simulink model "KVHSerial03"  (R2013a)
settings: Solver=FixedStepDiscrete  StartTime=0.0  StopTime=inf  FixedStep=0.001  RelTol=1e-3
undefined symbols (not defined in the file or in its folder): Ground, m_XR17D15x, standard, XOFF, XON
libraries: speedgoatlib x26, xpcseriallib x13, simulink x3, xpclib x2
settings Model: BufferReuse=off  Creator=bgbuss  LastModifiedBy=bgbuss
settings DataIOCC: LimitDataPoints=off  SignalLoggingSaveFormat=ModelDataLogs
settings OptimizationCC: BlockReduction=off  OptimizeBlockIOStorage=off  BufferReuse=off  ExpressionFolding=off  ExpressionDepthLimit=2147483647  LocalBlockOutputs=off
settings DebuggingCC: UnderspecifiedInitializationDetection=Simplified  FcnCallInpInsideContextMsg=EnableAllAsWarning  StrictBusMsg=ErrorOnBusTreatedAsVector
settings HardwareCC: ProdIntDivRoundTo=Zero  ProdEndianess=LittleEndian  ProdHWDeviceType=Generic->32-bit x86 compatible
settings RTWCC: SystemTargetFile=xpctarget.tlc  TemplateMakefile=xpc_default_tmf  Description=xPC Target  ProcessScript=xpctarget_make_rtw_hook
settings xpcTargetCC: TargetFcnLib=ansi_tfl_table_tmw.mat  CodeReplacementLibrary=XPC_BLAS  ParMdlRefBuildCompliant=on  ConcurrentExecutionCompliant=on  CombineSignalStateStructs=off  MATLABClassNameForMDSCustomization=xpcAperiodicCustomization  GRTInterface=on  GenerateAllocFcn=off  RL32LogBufSizeModifier=10000000  xPCTaskExecutionProfile=off  xPCRL32EventNumber=5000  xPCisModelTimeout=off  xPCModelTimeoutSecs=10  xPCLoadParamSetFile=off  xPCConcurrentTasks=off  xPCEnableSFAnimation=off

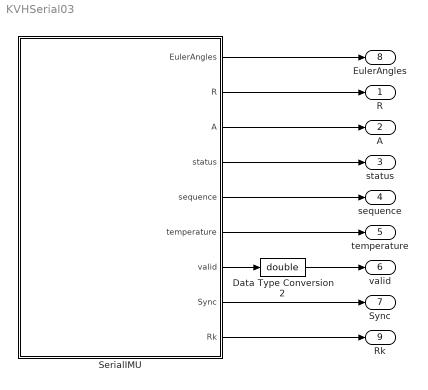
== system KVHSerial03 ==
  Data Type Conversion2 : DataTypeConversion  OutDataTypeStr=double
  SerialIMU : Subsystem
  R : Outport
  A : Outport  Port=2
  status : Outport  Port=3
  sequence : Outport  Port=4
  temperature : Outport  Port=5
  valid : Outport  Port=6
  Sync : Outport  Port=7
  EulerAngles : Outport  Port=8
  Rk : Outport  Port=9
  wires:
  SerialIMU/7(valid) -> Data Type Conversion2/1
  SerialIMU/3(A) -> A/1
  SerialIMU/2(R) -> R/1
  SerialIMU/4(status) -> status/1
  SerialIMU/5(sequence) -> sequence/1
  SerialIMU/6(temperature) -> temperature/1
  SerialIMU/8(Sync) -> Sync/1
  SerialIMU/1(EulerAngles) -> EulerAngles/1
  SerialIMU/9(Rk) -> Rk/1
  Data Type Conversion2/1 -> valid/1

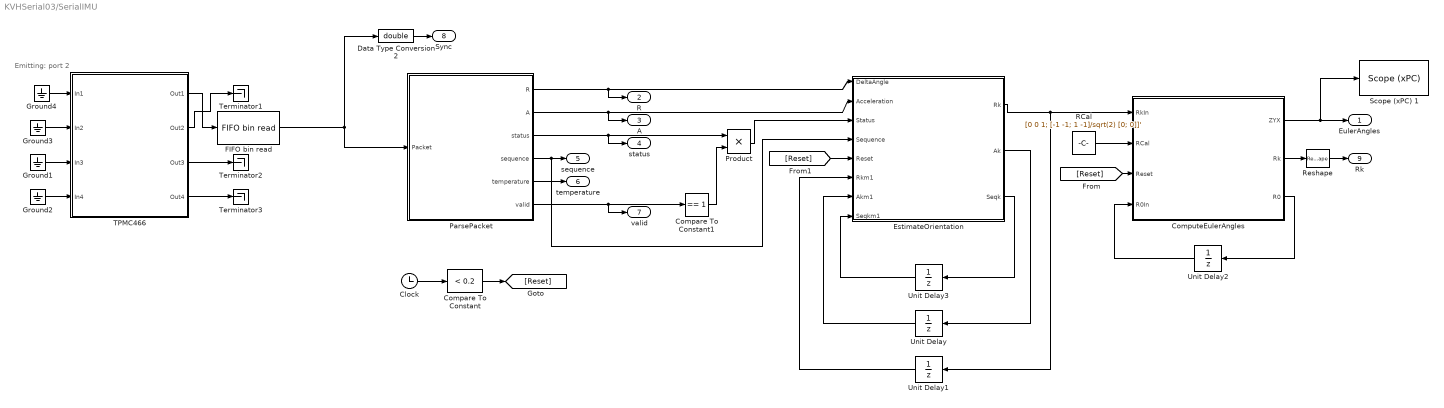
== system KVHSerial03/SerialIMU ==
  note: Emitting: port 2
  Clock : Clock
  Compare To Constant : simulink/Logic and Bit Operations/Compare To Constant  relop=<  const=0.2  OutDataTypeStr=uint8
  Compare To Constant1 : simulink/Logic and Bit Operations/Compare To Constant  relop===  const=1  OutDataTypeStr=uint8
  ComputeEulerAngles : MATLAB Function  TreatAsAtomicUnit=on
  Data Type Conversion2 : DataTypeConversion  OutDataTypeStr=double
  EstimateOrientation : MATLAB Function  TreatAsAtomicUnit=on
  "FIFO bin read " : xpcseriallib/FIFO bin read   header={char([254 129 255 85])}  lengths=[36]  hold=Zero output if no new data  enable=off  maxsize=64  outputtype=8 bit uint null terminated  sampletime=0.001
  Ground{1..4} (4 alike) : Ground
  ParsePacket : Subsystem
  Product : Product  RndMeth=Zero
  RCal : Constant  Value=[0 0 1; [-1 -1; 1 -1]/sqrt(2) [0; 0]]'
  Reshape : Reshape
  Scope (xPC) 1 : xpclib/Misc./Scope (xPC)   scopeno=1  scopetype=Target  autostart=on  viewmode=Graphical rolling  formatstr='%15.6f'  grid=on  ylimits=[-pi pi]  nosamples=500  noprepostsamples=0  interleave=10  triggermode=FreeRun  triggersignal=1  trigsignalfromport=off  triggerlevel=0.0  triggerslope=Either  triggerscope=1  triggersample=0  filename=data.dat  mode=Lazy  writesize=512  autorestart=off  dynamicfilemode=off  maxwritefilesize=512*1024^2
  TPMC466 : Subsystem  AncestorBlock=speedgoatlib/IO503/TPMC466  InitFcn=m_XR17D15x(3);  mask(RS232 Send Receive){group=Basic Setup, port=1, irqnum=9, slot=-1, transceiver1=RS422, standard1=on, baud1=921600, bauddivisor1=1, sampling1=16x (standard), prescale1=off, parity1=None, ndata1=8, nstop1=1, rlevel1=1, hwmode1=none, swmode1=none, xonchar1=17, xoffchar1=19, rs485auto1=off, rs485delay1=1, xmtfifosize1=1024, xmtdatatype1=8 bit uint null terminated, rcvfifosize1=1024, transceiver2=RS485 half-duplex, standard2=on, baud2=2764800, bauddivisor2=1, sampling2=16x (standard), prescale2=off, parity2=None, ndata2=8, nstop2=1, rlevel2=quarter full (16), hwmode2=none, swmode2=XON/XOFF, xonchar2=17, xoffchar2=19, rs485auto2=on, rs485delay2=1, xmtfifosize2=1024, xmtdatatype2=8 bit uint null terminated, rcvfifosize2=1024, transceiver3=RS485 half-duplex, standard3=on, baud3=115200, bauddivisor3=1, sampling3=16x (standard), prescale3=off, parity3=None, ndata3=8, nstop3=1, rlevel3=half full (32), hwmode3=none, swmode3=none, xonchar3=17, xoffchar3=19, rs485auto3=off, rs485delay3=0, xmtfifosize3=1024, xmtdatatype3=8 bit uint null terminated, rcvfifosize3=1024, transceiver4=RS485 half-duplex, standard4=on, baud4=115200, bauddivisor4=1, sampling4=16x (standard), prescale4=off, parity4=None, ndata4=8, nstop4=1, rlevel4=half full (32), hwmode4=none, swmode4=none, xonchar4=17, xoffchar4=19, rs485auto4=off, rs485delay4=0, xmtfifosize4=1024, xmtdatatype4=8 bit uint null terminated, rcvfifosize4=1024}
      mask prompts: group "Parameter group:"; port "Port to modify:"; irqnum "IRQ number:"; slot "PCI slot (-1: autosearch):"; transceiver1 "Transceiver setup:"; standard1 "Use standard baud rates (16x, no prescaling)"; baud1 "Standard baud rate:"; bauddivisor1 "Baud rate divisor (non-standard baud rates):"; sampling1 "Sampling rate (non-standard baud rates):"; prescale1 "Prescale by 4 (non-standard baud rates)"; parity1 "Parity:"; ndata1 "Data bits:"; nstop1 "Stop bits:"; rlevel1 "Receive FIFO interrupt level:"; hwmode1 "Hardware handshake:"; swmode1 "Software handshake:"; xonchar1 "XON character:"; xoffchar1 "XOFF character:"; rs485auto1 "RS485 auto turnaround:"; rs485delay1 "RS485 turnaround delay [0,15]"; xmtfifosize1 "Transmit software FIFO size:"; xmtdatatype1 "Transmit FIFO data type:"; rcvfifosize1 "Receive software FIFO size:"; transceiver2 "Transceiver setup:"; standard2 "Use standard baud rates (16x, no prescaling)"; baud2 "Standard baud rate:"; bauddivisor2 "Baud rate divisor (non-standard baud rates):"; sampling2 "Sampling rate (non-standard baud rates):"; prescale2 "Prescale by 4 (non-standard baud rates)"; parity2 "Parity:"; ndata2 "Data bits:"; nstop2 "Stop bits:"; rlevel2 "Receive FIFO interrupt level:"; hwmode2 "Hardware handshake:"; swmode2 "Software handshake:"; xonchar2 "XON character:"; xoffchar2 "XOFF character:"; rs485auto2 "RS485 auto turnaround:"; rs485delay2 "RS485 turnaround delay [0,15]"; xmtfifosize2 "Transmit software FIFO size:"; xmtdatatype2 "Transmit FIFO data type:"; rcvfifosize2 "Receive software FIFO size:"; transceiver3 "Transceiver setup:"; standard3 "Use standard baud rates (16x, no prescaling)"; baud3 "Standard baud rate:"; bauddivisor3 "Baud rate divisor (non-standard baud rates):"; sampling3 "Sampling rate (non-standard baud rates):"; prescale3 "Prescale by 4 (non-standard baud rates)"; parity3 "Parity:"; ndata3 "Data bits:"; nstop3 "Stop bits:"; rlevel3 "Receive FIFO interrupt level:"; hwmode3 "Hardware handshake:"; swmode3 "Software handshake:"; xonchar3 "XON character:"; xoffchar3 "XOFF character:"; rs485auto3 "RS485 auto turnaround:"; rs485delay3 "RS485 turnaround delay [0,15]"; xmtfifosize3 "Transmit software FIFO size:"; xmtdatatype3 "Transmit FIFO data type:"; rcvfifosize3 "Receive software FIFO size:"; transceiver4 "Transceiver setup:"; standard4 "Use standard baud rates (16x, no prescaling)"; baud4 "Standard baud rate:"; bauddivisor4 "Baud rate divisor (non-standard baud rates):"; sampling4 "Sampling rate (non-standard baud rates):"; prescale4 "Prescale by 4 (non-standard baud rates)"; parity4 "Parity:"; ndata4 "Data bits:"; nstop4 "Stop bits:"; rlevel4 "Receive FIFO interrupt level:"; hwmode4 "Hardware handshake:"; swmode4 "Software handshake:"; xonchar4 "XON character:"; xoffchar4 "XOFF character:"; rs485auto4 "RS485 auto turnaround:"; rs485delay4 "RS485 turnaround delay [0,15]"; xmtfifosize4 "Transmit software FIFO size:"; xmtdatatype4 "Transmit FIFO data type:"; rcvfifosize4 "Receive software FIFO size:"
      mask help:
      | PMC521
      | Acromag
      | EIA/TIA-422B Send Receive Subsystem
      mask init:
      | brdslot = slot;
      | m_tews_XR17D15x(1, 4);
      mask Help: helpview(fullfile(docroot, 'mapfiles', 'xpc.map'), 'Commtech_Subsystem')
      mask TypeOptions group: Board Setup | Basic Setup | FIFO Setup
      mask Callback group: m_tews_XR17D15x(2, 4);
      mask TypeOptions port: 1 | 2 | 3 | 4
      mask Callback port: m_tews_XR17D15x(2, 4);
      mask TypeOptions transceiver1: RS232 (max 921.6kb/s) | RS422 | RS422 multidrop | RS485 full-duplex | RS485 half-duplex
      mask TypeOptions baud1: 2764800 | 1382400 | 921600 | 460800 | 230400 | 115200 | 57600 | 38400 | 19200 | 9600 | 4800 | 2400 | 1200 | 600 | 400
      mask TypeOptions sampling1: 8x | 16x (standard)
      mask TypeOptions parity1: None | Even | Odd | Mark | Space
      mask TypeOptions ndata1: 5 | 6 | 7 | 8
      mask TypeOptions nstop1: 1 | 2
      mask TypeOptions rlevel1: 1 | quarter full (16) | half full (32) | almost full (56)
      mask TypeOptions hwmode1: RTS/CTS | none
      mask TypeOptions swmode1: XON/XOFF | none
      mask TypeOptions xmtdatatype1: count+32 bit int | count+32 bit uint | count+16 bit int | count+16 bit uint | 8 bit int null terminated | 8 bit uint null terminated
      mask TypeOptions transceiver2: RS232 (max 921.6kb/s) | RS422 | RS422 multidrop | RS485 full-duplex | RS485 half-duplex
      mask TypeOptions baud2: 2764800 | 1382400 | 921600 | 460800 | 230400 | 115200 | 57600 | 38400 | 19200 | 9600 | 4800 | 2400 | 1200 | 600 | 400
      mask TypeOptions sampling2: 8x | 16x (standard)
      mask TypeOptions parity2: None | Even | Odd | Mark | Space
      mask TypeOptions ndata2: 5 | 6 | 7 | 8
      mask TypeOptions nstop2: 1 | 2
      mask TypeOptions rlevel2: 1 | quarter full (16) | half full (32) | almost full (56)
      mask TypeOptions hwmode2: RTS/CTS | none
      mask TypeOptions swmode2: XON/XOFF | none
      mask TypeOptions xmtdatatype2: count+32 bit int | count+32 bit uint | count+16 bit int | count+16 bit uint | 8 bit int null terminated | 8 bit uint null terminated
      mask TypeOptions transceiver3: RS232 (max 921.6kb/s) | RS422 | RS422 multidrop | RS485 full-duplex | RS485 half-duplex
      mask TypeOptions baud3: 2764800 | 1382400 | 921600 | 460800 | 230400 | 115200 | 57600 | 38400 | 19200 | 9600 | 4800 | 2400 | 1200 | 600 | 400
      mask TypeOptions sampling3: 8x | 16x (standard)
      mask TypeOptions parity3: None | Even | Odd | Mark | Space
      mask TypeOptions ndata3: 5 | 6 | 7 | 8
      mask TypeOptions nstop3: 1 | 2
      mask TypeOptions rlevel3: 1 | quarter full (16) | half full (32) | almost full (56)
      mask TypeOptions hwmode3: RTS/CTS | none
      mask TypeOptions swmode3: XON/XOFF | none
      mask TypeOptions xmtdatatype3: count+32 bit int | count+32 bit uint | count+16 bit int | count+16 bit uint | 8 bit int null terminated | 8 bit uint null terminated
      mask TypeOptions transceiver4: RS232 (max 921.6kb/s) | RS422 | RS422 multidrop | RS485 full-duplex | RS485 half-duplex
      mask TypeOptions baud4: 2764800 | 1382400 | 921600 | 460800 | 230400 | 115200 | 57600 | 38400 | 19200 | 9600 | 4800 | 2400 | 1200 | 600 | 400
      mask TypeOptions sampling4: 8x | 16x (standard)
      mask TypeOptions parity4: None | Even | Odd | Mark | Space
      mask TypeOptions ndata4: 5 | 6 | 7 | 8
      mask TypeOptions nstop4: 1 | 2
      mask TypeOptions rlevel4: 1 | quarter full (16) | half full (32) | almost full (56)
      mask TypeOptions hwmode4: RTS/CTS | none
      mask TypeOptions swmode4: XON/XOFF | none
      mask TypeOptions xmtdatatype4: count+32 bit int | count+32 bit uint | count+16 bit int | count+16 bit uint | 8 bit int null terminated | 8 bit uint null terminated
      mask Display:
      | disp('TEWS\nTPMC466\nRS232/422/485\nSend\nReceive');
      | port_label( 'input', 1, 'XMT1' );
      | port_label( 'input', 2, 'XMT2' );
      | port_label( 'input', 3, 'XMT3' );
      | port_label( 'input', 4, 'XMT4' );
      | 
      | port_label( 'output', 1, 'FIFO1' );
      | port_label( 'output', 2, 'FIFO2' );
      | port_label( 'output', 3, 'FIFO3' );
      | port_label( 'output', 4, 'FIFO4' );
  Terminator1 : Terminator
  Terminator2 : Terminator
  Terminator3 : Terminator
  Unit Delay : UnitDelay  InitialCondition=[0; 0; 0]  SampleTime=-1
  Unit Delay1 : UnitDelay  InitialCondition=zeros(3,3)  SampleTime=-1
  Unit Delay2 : UnitDelay  InitialCondition=zeros(3,3)  SampleTime=-1
  Unit Delay3 : UnitDelay  SampleTime=-1
  EulerAngles : Outport
  R : Outport  Port=2
  A : Outport  Port=3
  status : Outport  Port=4
  sequence : Outport  Port=5
  temperature : Outport  Port=6
  valid : Outport  Port=7
  Sync : Outport  Port=8
  Rk : Outport  Port=9
  wires:
  ParsePacket/2(A) -> EstimateOrientation/2(Acceleration), A/1
  ParsePacket/1(R) -> EstimateOrientation/1(DeltaAngle), R/1
  ParsePacket/3(status) -> status/1, Product/1
  ParsePacket/4(sequence) -> EstimateOrientation/4(Sequence), sequence/1
  ParsePacket/5(temperature) -> temperature/1
  "FIFO bin read "/1 -> ParsePacket/1(Packet), Data Type Conversion2/1
  ParsePacket/6(valid) -> valid/1, Compare To Constant1/1
  Data Type Conversion2/1 -> Sync/1
  EstimateOrientation/2(Ak) -> Unit Delay/1
  Unit Delay/1 -> EstimateOrientation/7(Akm1)
  EstimateOrientation/1(Rk) -> Unit Delay1/1, ComputeEulerAngles/1(RkIn)
  Unit Delay1/1 -> EstimateOrientation/6(Rkm1)
  [Reset] -> EstimateOrientation/5(Reset)
  RCal/1 -> ComputeEulerAngles/2(RCal)
  Unit Delay2/1 -> ComputeEulerAngles/4(R0In)
  ComputeEulerAngles/1(ZYX) -> Scope (xPC) 1/1, EulerAngles/1
  ComputeEulerAngles/3(R0) -> Unit Delay2/1
  ComputeEulerAngles/2(Rk) -> Reshape/1
  [Reset] -> ComputeEulerAngles/3(Reset)
  Clock/1 -> Compare To Constant/1
  Compare To Constant/1 -> [Reset]
  Reshape/1 -> Rk/1
  Product/1 -> EstimateOrientation/3(Status)
  Compare To Constant1/1 -> Product/2
  Ground4/1 -> TPMC466/1(In1)
  Ground3/1 -> TPMC466/2(In2)
  Ground1/1 -> TPMC466/3(In3)
  Ground2/1 -> TPMC466/4(In4)
  TPMC466/3(Out3) -> Terminator2/1
  TPMC466/4(Out4) -> Terminator3/1
  TPMC466/1(Out1) -> "FIFO bin read "/1
  TPMC466/2(Out2) -> Terminator1/1
  EstimateOrientation/3(Seqk) -> Unit Delay3/1
  Unit Delay3/1 -> EstimateOrientation/8(Seqkm1)

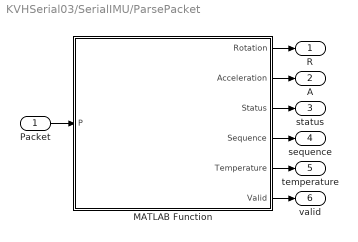
== system KVHSerial03/SerialIMU/ParsePacket ==
  Packet : Inport
  MATLAB Function : MATLAB Function  TreatAsAtomicUnit=on
  R : Outport
  A : Outport  Port=2
  status : Outport  Port=3
  sequence : Outport  Port=4
  temperature : Outport  Port=5
  valid : Outport  Port=6
  wires:
  MATLAB Function/1(Rotation) -> R/1
  MATLAB Function/2(Acceleration) -> A/1
  MATLAB Function/3(Status) -> status/1
  Packet/1 -> MATLAB Function/1(P)
  MATLAB Function/4(Sequence) -> sequence/1
  MATLAB Function/5(Temperature) -> temperature/1
  MATLAB Function/6(Valid) -> valid/1

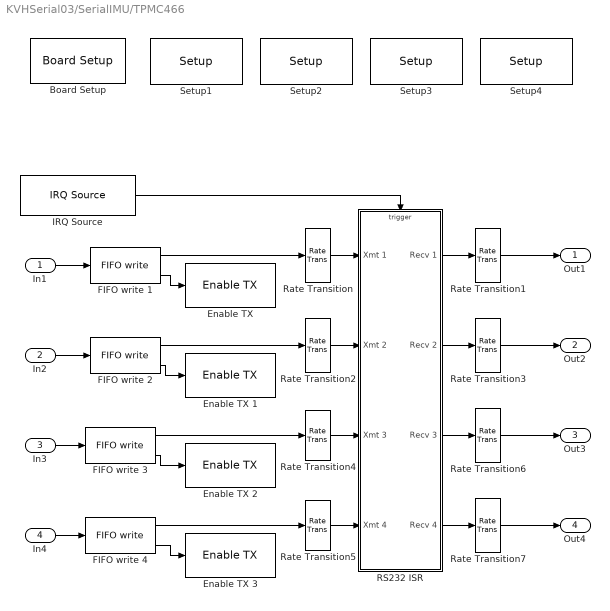
== system KVHSerial03/SerialIMU/TPMC466 ==
  In1 : Inport
  In2 : Inport  Port=2
  In3 : Inport  Port=3
  In4 : Inport  Port=4
  Board Setup : speedgoatlib/IO503/TEWS TPMC466 Internal blocks/Board Setup  irqnum=9  slot=brdslot
  "Enable TX " : speedgoatlib/IO503/TEWS TPMC466 Internal blocks/Enable TX   port=1  slot=brdslot
  Enable TX 1 : speedgoatlib/IO503/TEWS TPMC466 Internal blocks/Enable TX   port=2  slot=brdslot
  Enable TX 2 : speedgoatlib/IO503/TEWS TPMC466 Internal blocks/Enable TX   port=3  slot=brdslot
  Enable TX 3 : speedgoatlib/IO503/TEWS TPMC466 Internal blocks/Enable TX   port=4  slot=brdslot
  FIFO write 1 : xpcseriallib/FIFO write   size=1024  inputtype=8 bit uint null terminated  present=on  sampletime=-1  id=XMT channel 1, IRQ 9
  FIFO write 2 : xpcseriallib/FIFO write   size=1024  inputtype=8 bit uint null terminated  present=on  sampletime=-1  id=XMT channel 2, IRQ 9
  FIFO write 3 : xpcseriallib/FIFO write   size=1024  inputtype=8 bit uint null terminated  present=on  sampletime=-1  id=XMT channel 3, IRQ 9
  FIFO write 4 : xpcseriallib/FIFO write   size=1024  inputtype=8 bit uint null terminated  present=on  sampletime=-1  id=XMT channel 4, IRQ 9
  IRQ Source : xpclib/Asynchronous Event/IRQ Source  irqNo=9  preempt=off  b_type=None/Other  slot=brdslot
  RS232 ISR : Subsystem  TreatAsAtomicUnit=on  mask(RS232 ISR){slot=brdslot}
      mask help:
      | PMC521
      | Acromag
      | Interrupt Service Routine
      mask init:
      | subslot = slot;
      mask Display:
      | disp('PMC521\nAcromag\nISR');
      | port_label('input', 1, 'XMT1');
      | port_label('input', 2, 'XMT2');
      | port_label('input', 3, 'XMT3');
      | port_label('input', 4, 'XMT4');
      | port_label('input', 5, 'XMT5');
      | port_label('input', 6, 'XMT6');
      | port_label('input', 7, 'XMT7');
      | port_label('input', 8, 'XMT8');
      | port_label('output', 1, 'RCV1');
      | port_label('output', 2, 'RCV2');
      | port_label('output', 3, 'RCV3');
      | port_label('output', 4, 'RCV4');
      | port_label('output', 5, 'RCV5');
      | port_label('output', 6, 'RCV6');
      | port_label('output', 7, 'RCV7');
      | port_label('output', 8, 'RCV8');
  Rate Transition{,2,4..5} (4 alike) : RateTransition  Integrity=off  Deterministic=off
  Rate Transition{1,3,6..7} (4 alike) : RateTransition  Integrity=off  Deterministic=off  OutPortSampleTime=0
  Setup1 : speedgoatlib/IO503/TEWS TPMC466 Internal blocks/Setup   port=1  transceiver=RS422  standard=on  baudrate=921600  bauddivisor=1  mode8x=16x (standard)  prescale=off  width=8  nstop=1  parity=None  rlevel=1  ctsmode=none  xonoff=none  xon=17  xoff=19  rs485mode=off  rs485delay=1  slot=brdslot
  Setup2 : speedgoatlib/IO503/TEWS TPMC466 Internal blocks/Setup   port=2  transceiver=RS485 half-duplex  standard=on  baudrate=2764800  bauddivisor=1  mode8x=16x (standard)  prescale=off  width=8  nstop=1  parity=None  rlevel=quarter full (16)  ctsmode=none  xonoff=XON/XOFF  xon=17  xoff=19  rs485mode=on  rs485delay=1  slot=brdslot
  Setup3 : speedgoatlib/IO503/TEWS TPMC466 Internal blocks/Setup   port=3  transceiver=RS485 half-duplex  standard=on  baudrate=115200  bauddivisor=1  mode8x=16x (standard)  prescale=off  width=8  nstop=1  parity=None  rlevel=half full (32)  ctsmode=none  xonoff=none  xon=17  xoff=19  rs485mode=off  rs485delay=0  slot=brdslot
  Setup4 : speedgoatlib/IO503/TEWS TPMC466 Internal blocks/Setup   port=4  transceiver=RS485 half-duplex  standard=on  baudrate=115200  bauddivisor=1  mode8x=16x (standard)  prescale=off  width=8  nstop=1  parity=None  rlevel=half full (32)  ctsmode=none  xonoff=none  xon=17  xoff=19  rs485mode=off  rs485delay=0  slot=brdslot
  Out1 : Outport
  Out2 : Outport  Port=2
  Out3 : Outport  Port=3
  Out4 : Outport  Port=4
  wires:
  RS232 ISR/4(Recv 4) -> Rate Transition7/1
  RS232 ISR/3(Recv 3) -> Rate Transition6/1
  Rate Transition7/1 -> Out4/1
  Rate Transition6/1 -> Out3/1
  Rate Transition5/1 -> RS232 ISR/4(Xmt 4)
  Rate Transition4/1 -> RS232 ISR/3(Xmt 3)
  FIFO write 4/1 -> Rate Transition5/1
  In4/1 -> FIFO write 4/1
  FIFO write 4/2 -> Enable TX 3/1
  FIFO write 3/1 -> Rate Transition4/1
  In3/1 -> FIFO write 3/1
  FIFO write 3/2 -> Enable TX 2/1
  Rate Transition1/1 -> Out1/1
  Rate Transition3/1 -> Out2/1
  Rate Transition/1 -> RS232 ISR/1(Xmt 1)
  Rate Transition2/1 -> RS232 ISR/2(Xmt 2)
  FIFO write 1/2 -> "Enable TX "/1
  IRQ Source/1 -> RS232 ISR/Trigger
  RS232 ISR/1(Recv 1) -> Rate Transition1/1
  RS232 ISR/2(Recv 2) -> Rate Transition3/1
  FIFO write 1/1 -> Rate Transition/1
  In1/1 -> FIFO write 1/1
  FIFO write 2/1 -> Rate Transition2/1
  In2/1 -> FIFO write 2/1
  FIFO write 2/2 -> Enable TX 1/1

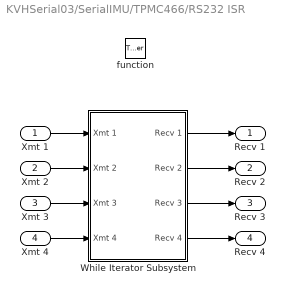
== system KVHSerial03/SerialIMU/TPMC466/RS232 ISR ==
  Xmt 1 : Inport
  Xmt 2 : Inport  Port=2
  Xmt 3 : Inport  Port=3
  Xmt 4 : Inport  Port=4
  function : TriggerPort  TriggerType=function-call
  While Iterator Subsystem : Subsystem  TreatAsAtomicUnit=on
  Recv 1 : Outport  SourceOfInitialOutputValue=Input signal  InitialOutput=Ground
  Recv 2 : Outport  Port=2  SourceOfInitialOutputValue=Input signal  InitialOutput=uint32(0);
  Recv 3 : Outport  Port=3  SourceOfInitialOutputValue=Input signal  InitialOutput=uint32([0]);
  Recv 4 : Outport  Port=4  SourceOfInitialOutputValue=Input signal  InitialOutput=uint32([0]);
  wires:
  While Iterator Subsystem/4(Recv 4) -> Recv 4/1
  While Iterator Subsystem/3(Recv 3) -> Recv 3/1
  Xmt 4/1 -> While Iterator Subsystem/4(Xmt 4)
  Xmt 3/1 -> While Iterator Subsystem/3(Xmt 3)
  While Iterator Subsystem/2(Recv 2) -> Recv 2/1
  While Iterator Subsystem/1(Recv 1) -> Recv 1/1
  Xmt 2/1 -> While Iterator Subsystem/2(Xmt 2)
  Xmt 1/1 -> While Iterator Subsystem/1(Xmt 1)

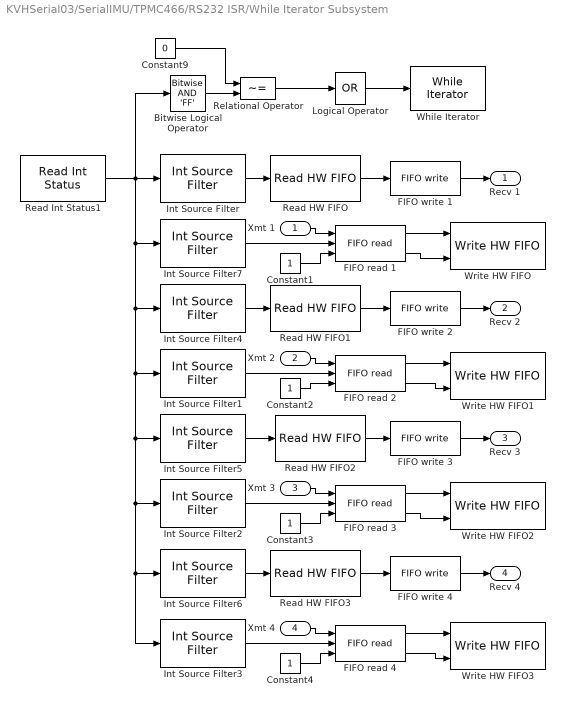
== system KVHSerial03/SerialIMU/TPMC466/RS232 ISR/While Iterator Subsystem ==
  Xmt 1 : Inport
  Xmt 2 : Inport  Port=2
  Xmt 3 : Inport  Port=3
  Xmt 4 : Inport  Port=4
  Bitwise Logical Operator : simulink/Logic and Bit Operations/Bitwise Operator  logicop=AND  UseBitMask=on  BitMask='FF'  BitMaskRealWorld=Stored Integer
  Constant{1..4} (4 alike) : Constant  OutDataTypeStr=uint32
  Constant9 : Constant  Value=0  OutDataTypeStr=uint32
  FIFO read {1..4} (4 alike) : xpcseriallib/FIFO read   maxsize=60  minsize=1  usedelimiter=off  delimiter=13  outputtype=count+32 bit uint  enable=on  enableout=on  sampletime=-1
  FIFO write 1 : xpcseriallib/FIFO write   size=1024  inputtype=count+32 bit uint  present=off  sampletime=-1  id=RCV channel 1, IRQ 9
  FIFO write 2 : xpcseriallib/FIFO write   size=1024  inputtype=count+32 bit uint  present=off  sampletime=-1  id=RCV channel 2, IRQ 9
  FIFO write 3 : xpcseriallib/FIFO write   size=1024  inputtype=count+32 bit uint  present=off  sampletime=-1  id=RCV channel 3, IRQ 9
  FIFO write 4 : xpcseriallib/FIFO write   size=1024  inputtype=count+32 bit uint  present=off  sampletime=-1  id=RCV channel 4, IRQ 9
  Int Source Filter : speedgoatlib/IO503/TEWS TPMC466 Internal blocks/Int Source Filter  port=1  value=Receive data
  Int Source Filter1 : speedgoatlib/IO503/TEWS TPMC466 Internal blocks/Int Source Filter  port=2  value=Transmitter empty
  Int Source Filter2 : speedgoatlib/IO503/TEWS TPMC466 Internal blocks/Int Source Filter  port=3  value=Transmitter empty
  Int Source Filter3 : speedgoatlib/IO503/TEWS TPMC466 Internal blocks/Int Source Filter  port=4  value=Transmitter empty
  Int Source Filter4 : speedgoatlib/IO503/TEWS TPMC466 Internal blocks/Int Source Filter  port=2  value=Receive data
  Int Source Filter5 : speedgoatlib/IO503/TEWS TPMC466 Internal blocks/Int Source Filter  port=3  value=Receive data
  Int Source Filter6 : speedgoatlib/IO503/TEWS TPMC466 Internal blocks/Int Source Filter  port=4  value=Receive data
  Int Source Filter7 : speedgoatlib/IO503/TEWS TPMC466 Internal blocks/Int Source Filter  port=1  value=Transmitter empty
  Logical Operator : Logic  Operator=OR  Inputs=1  AllPortsSameDT=off
  Read HW FIFO : speedgoatlib/IO503/TEWS TPMC466 Internal blocks/Read HW FIFO  port=1  flush=on  slot=subslot
  Read HW FIFO1 : speedgoatlib/IO503/TEWS TPMC466 Internal blocks/Read HW FIFO  port=2  flush=on  slot=subslot
  Read HW FIFO2 : speedgoatlib/IO503/TEWS TPMC466 Internal blocks/Read HW FIFO  port=3  flush=on  slot=subslot
  Read HW FIFO3 : speedgoatlib/IO503/TEWS TPMC466 Internal blocks/Read HW FIFO  port=4  flush=on  slot=subslot
  Read Int Status1 : speedgoatlib/IO503/TEWS TPMC466 Internal blocks/Read Int Status  slot=subslot
  Relational Operator : RelationalOperator  Operator=~=
  While Iterator : WhileIterator  MaxIters=65  WhileBlockType=do-while
  Write HW FIFO : speedgoatlib/IO503/TEWS TPMC466 Internal blocks/Write HW FIFO  port=1  slot=subslot
  Write HW FIFO1 : speedgoatlib/IO503/TEWS TPMC466 Internal blocks/Write HW FIFO  port=2  slot=subslot
  Write HW FIFO2 : speedgoatlib/IO503/TEWS TPMC466 Internal blocks/Write HW FIFO  port=3  slot=subslot
  Write HW FIFO3 : speedgoatlib/IO503/TEWS TPMC466 Internal blocks/Write HW FIFO  port=4  slot=subslot
  Recv 1 : Outport  SourceOfInitialOutputValue=Input signal  InitialOutput=uint32([0]);
  Recv 2 : Outport  Port=2  SourceOfInitialOutputValue=Input signal  InitialOutput=uint32([0]);
  Recv 3 : Outport  Port=3  SourceOfInitialOutputValue=Input signal  InitialOutput=uint32([0]);
  Recv 4 : Outport  Port=4  SourceOfInitialOutputValue=Input signal  InitialOutput=uint32([0]);
  wires:
  Read HW FIFO3/1 -> FIFO write 4/1
  FIFO write 4/1 -> Recv 4/1
  Read HW FIFO2/1 -> FIFO write 3/1
  FIFO write 3/1 -> Recv 3/1
  Int Source Filter6/1 -> Read HW FIFO3/1
  Int Source Filter5/1 -> Read HW FIFO2/1
  Constant3/1 -> FIFO read 3/3
  FIFO read 3/2 -> Write HW FIFO2/2
  FIFO read 3/1 -> Write HW FIFO2/1
  Xmt 3/1 -> FIFO read 3/1
  Int Source Filter2/1 -> FIFO read 3/2
  Constant2/1 -> FIFO read 2/3
  Constant1/1 -> FIFO read 1/3
  FIFO read 2/2 -> Write HW FIFO1/2
  FIFO read 1/2 -> Write HW FIFO/2
  FIFO read 1/1 -> Write HW FIFO/1
  FIFO read 2/1 -> Write HW FIFO1/1
  Xmt 2/1 -> FIFO read 2/1
  Int Source Filter1/1 -> FIFO read 2/2
  Read HW FIFO1/1 -> FIFO write 2/1
  FIFO write 2/1 -> Recv 2/1
  Int Source Filter4/1 -> Read HW FIFO1/1
  Xmt 1/1 -> FIFO read 1/1
  Int Source Filter7/1 -> FIFO read 1/2
  Read HW FIFO/1 -> FIFO write 1/1
  FIFO write 1/1 -> Recv 1/1
  Int Source Filter/1 -> Read HW FIFO/1
  Read Int Status1/1 -> Bitwise Logical Operator/1, Int Source Filter6/1, Int Source Filter3/1, Int Source Filter2/1, Int Source Filter5/1, Int Source Filter1/1, Int Source Filter4/1, Int Source Filter7/1, Int Source Filter/1
  Constant9/1 -> Relational Operator/1
  Bitwise Logical Operator/1 -> Relational Operator/2
  Relational Operator/1 -> Logical Operator/1
  Logical Operator/1 -> While Iterator/1
  Constant4/1 -> FIFO read 4/3
  FIFO read 4/2 -> Write HW FIFO3/2
  FIFO read 4/1 -> Write HW FIFO3/1
  Xmt 4/1 -> FIFO read 4/1
  Int Source Filter3/1 -> FIFO read 4/2

== matlab function KVHSerial03/SerialIMU/ComputeEulerAngles ==
  data: RkIn input; RCal input; Reset input; R0In input; ZYX output; Rk output; R0 output
function [ZYX, Rk, R0] = fcn(RkIn, RCal, Reset, R0In) %#codegen
    % Convert from IMU frame to robot frame and compute Euler angles. The
    % yaw angle is zeroed whenever (Reset) is true.
        
    if (Reset)
        % Compute the rotation matrix which zeros the initial yaw
        qT0 = M_to_ZYX(RkIn*RCal);
        R0  = Rz(-qT0(1));
    else
        R0 = R0In;
    end
    
    % Transform from IMU to robot frame and zero initial yaw
    Rk = R0*RkIn*RCal;
    
    % Convert Rk to ZYX Euler angles
    ZYX = M_to_ZYX(Rk);
end

function R = Rz(t)
    R = [cos(t) -sin(t) 0; sin(t) cos(t) 0; 0 0 1];
end

== matlab function KVHSerial03/SerialIMU/EstimateOrientation ==
  data: DeltaAngle input; Acceleration input; Status input; Sequence input; Reset input; Rk output; Rkm1 input; Akm1 input; Ak output; Seqkm1 input; Seqk output
function [Rk, Ak, Seqk] = fcn(DeltaAngle,Acceleration,Status,Sequence,Reset,Rkm1,Akm1,Seqkm1) %#codegen
    [Rk, Ak, Seqk] = estimateOrientation(DeltaAngle,Acceleration,Rkm1,Akm1,Status,Sequence,Seqkm1,Reset);
end

== matlab function KVHSerial03/SerialIMU/ParsePacket/MATLAB Function ==
  data: P input; Rotation output; Acceleration output; Status output; Sequence output; Temperature output; Valid output
function [Rotation,Acceleration,Status,Sequence,Temperature,Valid] = KVHParsePacket(P)
    %#codegen
    CMD = [254; 129; 255; 85]; %hex2dec(['FE';'81';'FF';'55']);
    
    Valid = false;
    if all(P(1:4) == CMD)
        Valid = kvhCheckCRC(P(1:36));
    end
    
    Rotation = parseSingle(P(5:16,:));
    Acceleration = parseSingle(P(17:28,:));
    Status = double(P(29));
    Sequence = double(P(30));
    Temperature = parseInt16(P(31:32));
end

function S = parseSingle(D)
    Stmp1 = uint32(reshape(D,4,[]));
    Stmp2 = 16777216*Stmp1(1,:) + 65536*Stmp1(2,:) + 256*Stmp1(3,:) + Stmp1(4,:);
    Stmp3 = typecast(Stmp2,'single');
    S = double(Stmp3');
end

function S = parseInt16(D)
    Stmp1 = uint16(reshape(D,2,[]));
    Stmp2 = 256*Stmp1(1,:) + Stmp1(2,:);
    S = double(Stmp2');
end
